simulink model "Main_Simulink"  (R2023b)
settings: Solver=FixedStepDiscrete  StartTime=0.0  StopTime=inf  FixedStep=0.001  RelTol=1e-3
undefined symbols (not defined in the file or in its folder): battery_builder_rtmsupport, gcbh, Initial_SOC
libraries: nesl_utility x118, pack_105s34p_structured_lib x105, fl_lib x14, ee_lib x7, dspstat3 x6, BatteryBalancing x1, deeplib x1
(part 2 of 10)

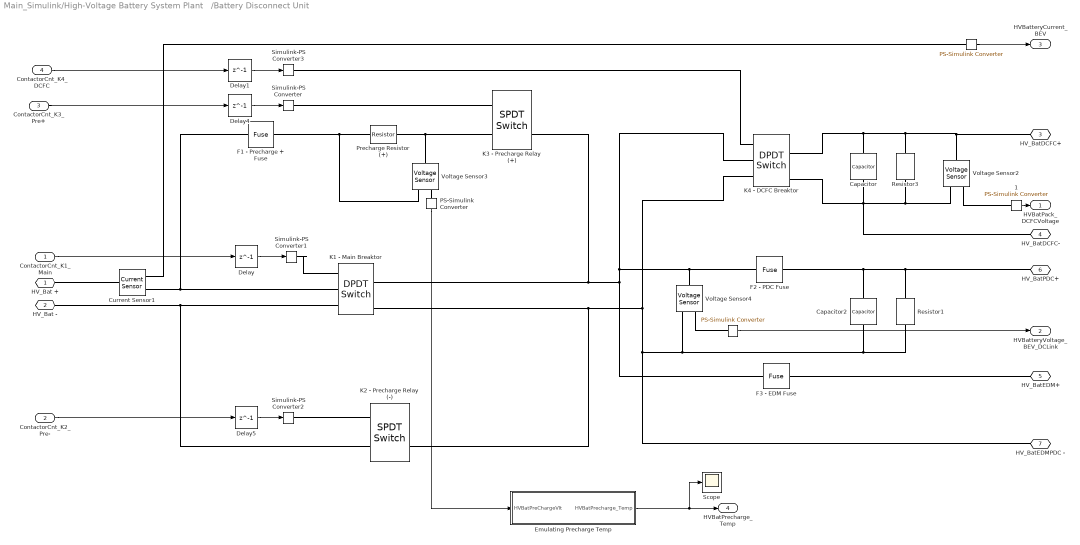
== system Main_Simulink/High-Voltage Battery System Plant   /Battery Disconnect Unit  ==
  ContactorCnt_K1_Main : Inport
  ContactorCnt_K2_Pre- : Inport  Port=2
  ContactorCnt_K3_Pre+ : Inport  Port=3
  ContactorCnt_K4_DCFC : Inport  Port=4
  "   " : nesl_utility/PS-Simulink Converter  PhysicalDomain=network_engine_domain  SubClassName=ps_output  LeftPortType=input  RightPortType=output  PseudoPeriodic=off  Frequencies=[]  VectorFormat=inherit  Unit=inherit  AffineConversion=off
  " " : nesl_utility/PS-Simulink Converter  PhysicalDomain=network_engine_domain  SubClassName=ps_output  LeftPortType=input  RightPortType=output  PseudoPeriodic=off  Frequencies=[]  VectorFormat=inherit  Unit=inherit  AffineConversion=off
  " 1" : nesl_utility/PS-Simulink Converter  PhysicalDomain=network_engine_domain  SubClassName=ps_output  LeftPortType=input  RightPortType=output  PseudoPeriodic=off  Frequencies=[]  VectorFormat=inherit  Unit=inherit  AffineConversion=off
  Capacitor : fl_lib/Electrical/Electrical Elements/Capacitor  c=750e-6 F  r=1e-6 Ohm  g=0 1/Ohm  i_specify=off  i_priority=None  i=0 A  i_nominal_specify=off  i_nominal_unit=A  i_nominal_value=1  v_specify=off  v_priority=None  v=0 V  v_nominal_specify=off  v_nominal_unit=V  v_nominal_value=1  vc_specify=off  vc_priority=High  vc=0 V  vc_nominal_specify=off  vc_nominal_unit=V  vc_nominal_value=1
  Capacitor2 : fl_lib/Electrical/Electrical Elements/Capacitor  c=750e-6 F  r=1e-6 Ohm  g=0 1/Ohm  i_specify=off  i_priority=None  i=0 A  i_nominal_specify=off  i_nominal_unit=A  i_nominal_value=1  v_specify=off  v_priority=None  v=0 V  v_nominal_specify=off  v_nominal_unit=V  v_nominal_value=1  vc_specify=off  vc_priority=High  vc=0 V  vc_nominal_specify=off  vc_nominal_unit=V  vc_nominal_value=1
  Current Sensor1 : fl_lib/Electrical/Electrical Sensors/Current Sensor
  Delay{,1,4..5} (4 alike) : Delay  DelayLength=1
  Emulating Precharge Temp : Subsystem
  F1 - Precharge + Fuse : ee_lib/Switches & Breakers/Fuse  prm=1  I_rated=600 A  melt_margin=1  T_fuse=0 s  I2t=1 A^2*s  I_vec=[1.9, 2, 2.5, 30] A  t_vec=[10000, 1, .3, .001] s  R_closed=0.01 Ohm  G_open=1e-8 1/Ohm  exposemeasurement=ee.enum.exposemeasurement.hidden
      settings: InternalSimscapePortConfiguration="{\"Bottom\":[],\"Left\":[{\"id\":\"p\",\"label\":\"\",\"type\":\"foundation.electrical.electrical\"}],\"Right\":[{\"id\":\"n\",\"label\":\"\",\"type\":\"foundation.electrical.electrical\"}],\"Top\":[]}"
  F2 - PDC Fuse : ee_lib/Switches & Breakers/Fuse  prm=1  I_rated=125 A  melt_margin=1  T_fuse=0 s  I2t=1 A^2*s  I_vec=[1.9, 2, 2.5, 30] A  t_vec=[10000, 1, .3, .001] s  R_closed=0.01 Ohm  G_open=1e-8 1/Ohm  exposemeasurement=ee.enum.exposemeasurement.hidden
      settings: InternalSimscapePortConfiguration="{\"Bottom\":[],\"Left\":[{\"id\":\"p\",\"label\":\"\",\"type\":\"foundation.electrical.electrical\"}],\"Right\":[{\"id\":\"n\",\"label\":\"\",\"type\":\"foundation.electrical.electrical\"}],\"Top\":[]}"
  F3 - EDM Fuse : ee_lib/Switches & Breakers/Fuse  prm=1  I_rated=600 A  melt_margin=1  T_fuse=0 s  I2t=1 A^2*s  I_vec=[1.9, 2, 2.5, 30] A  t_vec=[10000, 1, .3, .001] s  R_closed=0.01 Ohm  G_open=1e-8 1/Ohm  exposemeasurement=ee.enum.exposemeasurement.hidden
      settings: InternalSimscapePortConfiguration="{\"Bottom\":[],\"Left\":[{\"id\":\"p\",\"label\":\"\",\"type\":\"foundation.electrical.electrical\"}],\"Right\":[{\"id\":\"n\",\"label\":\"\",\"type\":\"foundation.electrical.electrical\"}],\"Top\":[]}"
  K1 - Main Breaktor : ee_lib/Switches & Breakers/DPDT Switch  R_closed=0.01 Ohm  G_open=1e-6 S  Threshold=0.5 V  Width=0 V  model_dynamics=0  t_on=1e-3 s  t_off=1e-3 s  initial_vT=0 V
      settings: InternalSimscapePortConfiguration="{\"Bottom\":[],\"Left\":[{\"id\":\"vT\",\"label\":\"vT\",\"type\":\"input\"},{\"id\":\"p1\",\"label\":\"\",\"type\":\"foundation.electrical.electrical\"},{\"id\":\"p2\",\"label\":\"\",\"type\":\"foundation.electrical.electrical\"}],\"Right\":[{\"id\":\"n11\",\"label\":\"\",\"type\":\"foundation.electrical.electrical\"},{\"id\":\"n12\",\"label\":\"\",\"type\":\"foundation.electrical.electrical\"},{\"id\":\"n21\",\"label\":\"\",\"type\":\"foundation.electrical.electrical\"},{\"id\":\"n22\",\"label\":\"\",\"type\":\"foundation.electrical.electrical\"}],\"Top\":[]}"
  K2 - Precharge Relay (-) : ee_lib/Switches & Breakers/SPDT Switch  R_closed=0.01 Ohm  G_open=1e-6 S  Threshold=0.5 V  Width=0 V  model_dynamics=0  t_on=1e-3 s  t_off=1e-3 s  initial_vT=0 V
  K3 - Precharge Relay (+) : ee_lib/Switches & Breakers/SPDT Switch  R_closed=0.01 Ohm  G_open=1e-6 S  Threshold=0.5 V  Width=0 V  model_dynamics=0  t_on=1e-3 s  t_off=1e-3 s  initial_vT=0 V
  K4 - DCFC Breaktor : ee_lib/Switches & Breakers/DPDT Switch  R_closed=0.01 Ohm  G_open=1e-6 S  Threshold=0.5 V  Width=0 V  model_dynamics=0  t_on=1e-3 s  t_off=1e-3 s  initial_vT=0 V
      settings: InternalSimscapePortConfiguration="{\"Bottom\":[],\"Left\":[{\"id\":\"vT\",\"label\":\"vT\",\"type\":\"input\"},{\"id\":\"p1\",\"label\":\"\",\"type\":\"foundation.electrical.electrical\"},{\"id\":\"p2\",\"label\":\"\",\"type\":\"foundation.electrical.electrical\"}],\"Right\":[{\"id\":\"n11\",\"label\":\"\",\"type\":\"foundation.electrical.electrical\"},{\"id\":\"n12\",\"label\":\"\",\"type\":\"foundation.electrical.electrical\"},{\"id\":\"n21\",\"label\":\"\",\"type\":\"foundation.electrical.electrical\"},{\"id\":\"n22\",\"label\":\"\",\"type\":\"foundation.electrical.electrical\"}],\"Top\":[]}"
  PS-Simulink Converter : nesl_utility/PS-Simulink Converter  PhysicalDomain=network_engine_domain  SubClassName=ps_output  LeftPortType=input  RightPortType=output  PseudoPeriodic=off  Frequencies=[]  VectorFormat=inherit  Unit=inherit  AffineConversion=off
  Precharge Resistor (+) : fl_lib/Electrical/Electrical Elements/Resistor  R=25 Ohm  i_specify=off  i_priority=None  i=0 A  i_nominal_specify=off  i_nominal_unit=A  i_nominal_value=1  v_specify=off  v_priority=None  v=0 V  v_nominal_specify=off  v_nominal_unit=V  v_nominal_value=1
  Resistor1 : fl_lib/Electrical/Electrical Elements/Resistor  R=40 kOhm  i_specify=off  i_priority=None  i=0 A  i_nominal_specify=off  i_nominal_unit=A  i_nominal_value=1  v_specify=off  v_priority=None  v=0 V  v_nominal_specify=off  v_nominal_unit=V  v_nominal_value=1
  Resistor3 : fl_lib/Electrical/Electrical Elements/Resistor  R=40 kOhm  i_specify=off  i_priority=None  i=0 A  i_nominal_specify=off  i_nominal_unit=A  i_nominal_value=1  v_specify=off  v_priority=None  v=0 V  v_nominal_specify=off  v_nominal_unit=V  v_nominal_value=1
  Scope : Scope
  Simulink-PS Converter{,1..3} (4 alike) : nesl_utility/Simulink-PS Converter  PhysicalDomain=network_engine_domain  SubClassName=ps_input  LeftPortType=input  RightPortType=output  PseudoPeriodic=off  Frequencies=[]  NoiseDistribution=none  NoiseParameters=[]  Unit=1  AffineConversion=off  FilteringAndDerivatives=provide  SimscapeFilterOrder=1  InputFilterTimeConstant=0.001  UdotUserProvided=0
  Voltage Sensor2 : fl_lib/Electrical/Electrical Sensors/Voltage Sensor
  Voltage Sensor3 : fl_lib/Electrical/Electrical Sensors/Voltage Sensor
  Voltage Sensor4 : fl_lib/Electrical/Electrical Sensors/Voltage Sensor
  "HV_Bat + " : PMIOPort  Side=Left
  HV_Bat - : PMIOPort  Port=2  Side=Left
  HV_BatDCFC+ : PMIOPort  Port=3  Side=Right
  HV_BatDCFC- : PMIOPort  Port=4  Side=Right
  HV_BatEDM+ : PMIOPort  Port=5  Side=Right
  HV_BatPDC+ : PMIOPort  Port=6  Side=Right
  HV_BatEDMPDC - : PMIOPort  Port=7  Side=Right
  HVBatPack_DCFCVoltage : Outport
  HVBatteryVoltage_BEV_DCLink : Outport  Port=2
  HVBatteryCurrent_BEV : Outport  Port=3
  HVBatPrecharge_Temp : Outport  Port=4
  wires:
  Delay1/1 -> Simulink-PS Converter3/1
  " 1"/1 -> HVBatPack_DCFCVoltage/1
  Delay5/1 -> Simulink-PS Converter2/1
  Delay4/1 -> Simulink-PS Converter/1
  "   "/1 -> HVBatteryCurrent_BEV/1
  ContactorCnt_K2_Pre-/1 -> Delay5/1
  Delay/1 -> Simulink-PS Converter1/1
  ContactorCnt_K4_DCFC/1 -> Delay1/1
  ContactorCnt_K1_Main/1 -> Delay/1
  ContactorCnt_K3_Pre+/1 -> Delay4/1
  PS-Simulink Converter/1 -> Emulating Precharge Temp/1(HVBatPreChargeVlt)
  " "/1 -> HVBatteryVoltage_BEV_DCLink/1
  Emulating Precharge Temp/1(HVBatPrecharge_Temp) -> Scope/1, HVBatPrecharge_Temp/1
  connections:
  Resistor3/LConn1 -- Voltage Sensor2/LConn1 -- HV_BatDCFC+/RConn1 -- Capacitor/LConn1 -- K4 - DCFC Breaktor/RConn2
  Voltage Sensor3/LConn1 -- K3 - Precharge Relay (+)/LConn2 -- Precharge Resistor (+)/LConn1
  Voltage Sensor3/RConn2 -- Precharge Resistor (+)/RConn1 -- F1 - Precharge + Fuse/RConn1
  Capacitor/RConn1 -- HV_BatDCFC-/RConn1 -- Voltage Sensor2/RConn2 -- Resistor3/RConn1 -- K4 - DCFC Breaktor/RConn4
  HV_BatEDM+/RConn1 -- F3 - EDM Fuse/LConn1
  Simulink-PS Converter1/RConn1 -- K1 - Main Breaktor/LConn1
  Voltage Sensor2/RConn1 -- " 1"/LConn1
  Resistor1/RConn1 -- Capacitor2/RConn1 -- HV_BatEDMPDC -/RConn1 -- K2 - Precharge Relay (-)/RConn2 -- K1 - Main Breaktor/RConn4 -- K4 - DCFC Breaktor/LConn3 -- Voltage Sensor4/RConn2
  "   "/LConn1 -- Current Sensor1/RConn1
  F2 - PDC Fuse/RConn1 -- Voltage Sensor4/LConn1 -- K3 - Precharge Relay (+)/RConn2 -- K1 - Main Breaktor/RConn2 -- F3 - EDM Fuse/RConn1 -- K4 - DCFC Breaktor/LConn2
  K2 - Precharge Relay (-)/LConn2 -- HV_Bat -/RConn1 -- K1 - Main Breaktor/LConn3
  K4 - DCFC Breaktor/LConn1 -- Simulink-PS Converter3/RConn1
  Simulink-PS Converter/RConn1 -- K3 - Precharge Relay (+)/LConn1
  Simulink-PS Converter2/RConn1 -- K2 - Precharge Relay (-)/LConn1
  F1 - Precharge + Fuse/LConn1 -- Current Sensor1/RConn2 -- K1 - Main Breaktor/LConn2
  PS-Simulink Converter/LConn1 -- Voltage Sensor3/RConn1
  Resistor1/LConn1 -- HV_BatPDC+/RConn1 -- F2 - PDC Fuse/LConn1 -- Capacitor2/LConn1
  Voltage Sensor4/RConn1 -- " "/LConn1
  "HV_Bat + "/RConn1 -- Current Sensor1/LConn1

== system Main_Simulink/High-Voltage Battery System Plant   /Charger//Load ==
  note: DC Fast Charging System
  note: Electric Drive Motor System
  note: Power Distribution Center System
  ChargeCurrentReq : Inport
  DrivingCurrentReq : Inport  Port=2
  ACChargeCurrentReq : Inport  Port=3
  Subsystem : Subsystem
  Subsystem1 : Subsystem
  Subsystem2 : Subsystem
  HV_BatDCFC+ : PMIOPort  Side=Left
  HV_BatDCFC- : PMIOPort  Port=2  Side=Left
  HV_BatEDM+ : PMIOPort  Port=3  Side=Left
  HV_BatPDC+ : PMIOPort  Port=4  Side=Left
  HV_BatEDMPDC - : PMIOPort  Port=5  Side=Left
  wires:
  ChargeCurrentReq/1 -> Subsystem/1(ChargeCurrentReq)
  DrivingCurrentReq/1 -> Subsystem1/1(DrivingCurrentReq)
  ACChargeCurrentReq/1 -> Subsystem2/1(ACChargeCurrentReq)
  connections:
  HV_BatDCFC+/RConn1 -- Subsystem/LConn1
  HV_BatDCFC-/RConn1 -- Subsystem/LConn2
  HV_BatEDMPDC -/RConn1 -- Subsystem2/LConn2 -- Subsystem1/LConn2
  HV_BatEDM+/RConn1 -- Subsystem1/LConn1
  HV_BatPDC+/RConn1 -- Subsystem2/LConn1

== system Main_Simulink/High-Voltage Battery System Plant   /ProMaster EV Battery Pack ==
  HVBatCellBalCmd : Inport
  Add : Sum
  Constant : Constant  Value=-273
  Constant1 : Constant  Value=25
  Constant2 : Constant  Value=25
  Delay : Delay  DelayLength=1
  Ground : fl_lib/Electrical/Electrical Elements/Electrical Reference
  "PS-Simulink " : nesl_utility/PS-Simulink Converter  PhysicalDomain=network_engine_domain  SubClassName=ps_output  LeftPortType=input  RightPortType=output  PseudoPeriodic=off  Frequencies=[]  VectorFormat=inherit  Unit=inherit  AffineConversion=off
  Pack1 : Subsystem  LoadFcn=battery_builder_rtmsupport('loadfcn',gcbh);
      settings: CopyFcn=battery_builder_rtmsupport('copyfcn',gcbh);  PreCopyFcn=battery_builder_rtmsupport('precopyfcn',gcbh);  PreDeleteFcn=battery_builder_rtmsupport('predeletefcn',gcbh);  PortSchema="{\"entries\":[{\"content\":{\"sides\":[{\"content\":{\"connectorIds\":[\"LConn1\"]},\"type\":\"ConnectorPlacement.EquallySpacedRectSide\",\"uuid\":\"64cec01f-33b3-4096-a4b7-6ded1472655c\"},{\"content\":{\"connectorIds\":[\"RConn1\"],\"side\":\"RIGHT\"},\"type\":\"ConnectorPlacement.EquallySpacedRectSide\",\"uuid\":\"f81a09ba-8909-4ce0-8a1f-4d13f5ea5620\"},{\"content\":{\"connectorIds\":[\"In1\"],\"side\":\"TOP\"},\"type\":\"ConnectorPlacement.EquallySpacedRectSide\",\"uuid\":\"a1cde63b-8eec-4d12-9d86-d553f5222491\"},{\"content\":{\"connectorIds\":[\"Out1\",\"Out2\",\"Out3\",\"Out4\",\"Out5\",\"Out6\",\"Out7\"],\"side\":\"BOTTOM\"},\"type\":\"ConnectorPlacement.EquallySpacedRectSide\",\"uuid\":\"7a252ceb-0eb8-4c98-af2a-dfdb6d4be7fd\"}]},\"type\":\"ConnectorPlacement.EquallySpacedConnector\",\"uuid\":\"c86ab74f-be26-4544-b601-79f59a4b6fde\"}],\"packageUris\":[\"http://schema.mathworks.com/mf0/Connector/R2020b\"],\"version\":\"1.0\"}"
      mask Display: image('$imagefile')
  Solver Configuration : nesl_utility/Solver Configuration  PhysicalDomain=network_engine_domain  SubClassName=solver  LeftPortType=input  RightPortType=generic  Tones=[]  Harmonics=[]  SimulateNoise=off  Profile=off  UseLocalSampling=off  EnableSwitchedLinearOptims=on  FrequencyDomain=off  UseCCode=off  RelTol=0.001  AbsTol=0.001  MinStep=1e-09  ToWorkspace=off  RevertToSquareIcSolve=off  NumHomotopyIterations=100  PhasorMode=off  PhasorModeNumHarmonics=1  ConsistencySolver=NEWTON_XTOL_AFTER_FTOL  IndexReductionMethod=DerivativeReplacement  DoDC=off  ResidualTolerance=1e-09  ConsistencyTolSource=GLOBAL  ConsistencyAbsTol=0.001  ConsistencyRelTol=0.001  ConsistencyTolFactor=0.001  UseLocalSolver=on  LocalSolverChoice=NE_BACKWARD_EULER_ADVANCER  ResolveIndetEquations=on  FunctionEvalNumThread=1  LocalSolverSampleTime=0.001  DoFixedCost=on  MaxNonlinIter=3  MaxModeIter=2  ComputeImpulses=off  ImpulseIterations=2  LinearAlgebra=auto  LinearAlgebraNumThread=0  EquationFormulation=NE_TIME_EF  DelaysMemoryBudget=1024  AutomaticFiltering=off  FilteringTimeConstant=0.001  PartitionStorageMethod=AS_NEEDED  PartitionMemoryBudget=1024  PartitionMethod=ROBUST  MultibodyUseLocalSolver=off  MultibodyLocalSolverChoice=ODE1  MultibodyLocalSolverSampleTime=0.001
  Terminator{1..5} (5 alike) : Terminator
  Voltage Sensor : fl_lib/Electrical/Electrical Sensors/Voltage Sensor
  "HV Bat + " : PMIOPort  Side=Right
  HV Bat - : PMIOPort  Port=2  Side=Right
  HVBatteryVoltage_BEV : Outport
  HVBatCellVlt : Outport  Port=2
  HVBatCellTemp : Outport  Port=3
  HVBatClgInletTemp : Outport  Port=4
  HVBatClgIOutletTemp : Outport  Port=5
  wires:
  Pack1/2(iCell) -> Terminator4/1
  Pack1/5(socParallelAssembly) -> Terminator2/1
  Pack1/1(vCell) -> HVBatCellVlt/1
  "PS-Simulink "/1 -> HVBatteryVoltage_BEV/1
  HVBatCellBalCmd/1 -> Delay/1
  Pack1/3(numCyclesCell) -> Terminator1/1
  Pack1/7(vParallelAssembly) -> Terminator3/1
  Delay/1 -> Pack1/1(balancing)
  Constant1/1 -> HVBatClgInletTemp/1
  Constant2/1 -> HVBatClgIOutletTemp/1
  Pack1/6(temperatureCell) -> Add/1
  Add/1 -> HVBatCellTemp/1
  Constant/1 -> Add/2
  Pack1/4(socCell) -> Terminator5/1
  connections:
  Voltage Sensor/RConn2 -- Ground/LConn1 -- Solver Configuration/RConn1 -- Pack1/RConn1 -- HV Bat -/RConn1
  "HV Bat + "/RConn1 -- Voltage Sensor/LConn1 -- Pack1/LConn1
  Voltage Sensor/RConn1 -- "PS-Simulink "/LConn1

== system Main_Simulink/Battery Management System/State of Charge Estimation System/Creating bus element ==
  HvBatSOCcell : Inport
  Bus Creator : BusCreator  Inputs=105
  Demux : Demux  Outputs=105
  HVBatSOCcell : Outport
  wires:
  Demux/23 -> Bus Creator/23
  Demux/82 -> Bus Creator/82
  Demux/22 -> Bus Creator/22
  Demux/30 -> Bus Creator/30
  Demux/75 -> Bus Creator/75
  Demux/13 -> Bus Creator/13
  Demux/66 -> Bus Creator/66
  Demux/31 -> Bus Creator/31
  Demux/12 -> Bus Creator/12
  Demux/56 -> Bus Creator/56
  Demux/27 -> Bus Creator/27
  Demux/64 -> Bus Creator/64
  Demux/86 -> Bus Creator/86
  Demux/100 -> Bus Creator/100
  Demux/89 -> Bus Creator/89
  Demux/90 -> Bus Creator/90
  Demux/94 -> Bus Creator/94
  Demux/101 -> Bus Creator/101
  Demux/91 -> Bus Creator/91
  Demux/96 -> Bus Creator/96
  Demux/97 -> Bus Creator/97
  Demux/105 -> Bus Creator/105
  Demux/104 -> Bus Creator/104
  Demux/84 -> Bus Creator/84
  Demux/85 -> Bus Creator/85
  Demux/80 -> Bus Creator/80
  Demux/83 -> Bus Creator/83
  Demux/21 -> Bus Creator/21
  Demux/42 -> Bus Creator/42
  Demux/74 -> Bus Creator/74
  Demux/95 -> Bus Creator/95
  Demux/41 -> Bus Creator/41
  Demux/102 -> Bus Creator/102
  Demux/14 -> Bus Creator/14
  Demux/7 -> Bus Creator/7
  Demux/63 -> Bus Creator/63
  Demux/20 -> Bus Creator/20
  Demux/78 -> Bus Creator/78
  Demux/87 -> Bus Creator/87
  Demux/59 -> Bus Creator/59
  Demux/26 -> Bus Creator/26
  Demux/33 -> Bus Creator/33
  Demux/32 -> Bus Creator/32
  Demux/73 -> Bus Creator/73
  Demux/28 -> Bus Creator/28
  Demux/15 -> Bus Creator/15
  Demux/17 -> Bus Creator/17
  Demux/35 -> Bus Creator/35
  Demux/93 -> Bus Creator/93
  Demux/16 -> Bus Creator/16
  Demux/29 -> Bus Creator/29
  Demux/71 -> Bus Creator/71
  Demux/47 -> Bus Creator/47
  Demux/19 -> Bus Creator/19
  Demux/10 -> Bus Creator/10
  Demux/54 -> Bus Creator/54
  Demux/18 -> Bus Creator/18
  Demux/53 -> Bus Creator/53
  Demux/11 -> Bus Creator/11
  Demux/81 -> Bus Creator/81
  Demux/70 -> Bus Creator/70
  Demux/3 -> Bus Creator/3
  Demux/52 -> Bus Creator/52
  Demux/5 -> Bus Creator/5
  Demux/1 -> Bus Creator/1
  Demux/37 -> Bus Creator/37
  Demux/68 -> Bus Creator/68
  Demux/38 -> Bus Creator/38
  Demux/8 -> Bus Creator/8
  Demux/58 -> Bus Creator/58
  Demux/34 -> Bus Creator/34
  Demux/103 -> Bus Creator/103
  Demux/98 -> Bus Creator/98
  Demux/24 -> Bus Creator/24
  Demux/36 -> Bus Creator/36
  Demux/62 -> Bus Creator/62
  Demux/39 -> Bus Creator/39
  Demux/88 -> Bus Creator/88
  Demux/40 -> Bus Creator/40
  Demux/50 -> Bus Creator/50
  Demux/92 -> Bus Creator/92
  Demux/55 -> Bus Creator/55
  Demux/43 -> Bus Creator/43
  Demux/48 -> Bus Creator/48
  Demux/60 -> Bus Creator/60
  Demux/49 -> Bus Creator/49
  Demux/25 -> Bus Creator/25
  Demux/57 -> Bus Creator/57
  Demux/45 -> Bus Creator/45
  Demux/46 -> Bus Creator/46
  Demux/69 -> Bus Creator/69
  Demux/67 -> Bus Creator/67
  Demux/65 -> Bus Creator/65
  Demux/9 -> Bus Creator/9
  Demux/61 -> Bus Creator/61
  Demux/99 -> Bus Creator/99
  Demux/76 -> Bus Creator/76
  Demux/72 -> Bus Creator/72
  Demux/6 -> Bus Creator/6
  Demux/77 -> Bus Creator/77
  Demux/4 -> Bus Creator/4
  Demux/79 -> Bus Creator/79
  Bus Creator/1 -> HVBatSOCcell/1
  HvBatSOCcell/1 -> Demux/1
  Demux/2 -> Bus Creator/2
  Demux/44 -> Bus Creator/44
  Demux/51 -> Bus Creator/51

== system Main_Simulink/Battery Management System/State of Charge Estimation System/For Each Subsystem1 ==
  HVBatteryCurrent_BEV : Inport
  HVBatCellVlt : Inport  Port=2  Partition=on  PartitionDimension=1  PartitionWidth=1  PartitionOffset=0
  HVBatCellTemp : Inport  Port=3  Partition=on  PartitionDimension=1  PartitionWidth=1  PartitionOffset=0
  Data Type Conversion : DataTypeConversion  SaturateOnIntegerOverflow=off  RndMeth=Floor
  Discrete Filter : DiscreteFilter  Numerator=[0.003131764229193,0.003131764229193]  Denominator=[1,-0.993736471541615]
  Discrete Filter1 : DiscreteFilter  Numerator=[0.003131764229193,0.003131764229193]  Denominator=[1,-0.993736471541615]
  Discrete Filter2 : DiscreteFilter  Numerator=[0.003131764229193,0.003131764229193]  Denominator=[1,-0.993736471541615]
  For Each : ForEach  DisableCoverage=on
  Gain : Gain  Gain=100
  MATLAB Function8 : MATLAB Function  TreatAsAtomicUnit=on
  Mux : Mux
  Normalize block - Current : Subsystem
  Normalize block - Kalman Filter SoC : Subsystem
  Normalize block - Temperature : Subsystem
  Normalize block -Voltage : Subsystem
  Predict : deeplib/Predict  Network=Network from MAT-file  NetworkFunction=squeezenet  NetworkFilePath=C:\Users\mcmas\Downloads\bwc\ProMaster RAM EV Plant\EKF-FNN.mat  MiniBatchSize=128  InputDataFormats={'',''}  Predictions=on  Activations={}  ForceInterpretedSim=off  EnableDLNetwork=on
      link override "MLFB/ Demux ": Outputs=1
      link override "MLFB/ SFunction ": FunctionName=sf_sfun
      link override MLFB/in_1: Port=1
      link override MLFB/out_1_predict: Port=1
  Subsystem : Subsystem
  Transpose{,1..3} (4 alike) : Math  Operator=transpose
  HvBatSOCcell : Outport  ConcatenationDimension=1
  wires:
  HVBatCellTemp/1 -> Subsystem/3(Temperature), Discrete Filter2/1
  Gain/1 -> HvBatSOCcell/1
  Discrete Filter1/1 -> Normalize block -Voltage/1(Voltage)
  Data Type Conversion/1 -> Gain/1
  Discrete Filter/1 -> Normalize block - Current/1(Current)
  Normalize block - Current/1(Normalized current) -> Transpose/1
  Transpose3/1 -> Mux/4
  Normalize block - Kalman Filter SoC/1(Normalized State of Charge) -> Transpose3/1
  Transpose/1 -> Mux/1
  Discrete Filter2/1 -> Normalize block - Temperature/1(Temperature)
  Transpose2/1 -> Mux/3
  Mux/1 -> Predict/1
  Subsystem/1(SOC) -> Normalize block - Kalman Filter SoC/1(State of Charge)
  Normalize block - Temperature/1(Normalized temperature) -> Transpose2/1
  Predict/1 -> MATLAB Function8/1(SOC)
  HVBatCellVlt/1 -> Subsystem/2(Voltage), Discrete Filter1/1
  Normalize block -Voltage/1(Normalized voltage) -> Transpose1/1
  HVBatteryCurrent_BEV/1 -> Subsystem/1(Current), Discrete Filter/1
  Transpose1/1 -> Mux/2
  MATLAB Function8/1(SOC_Output) -> Data Type Conversion/1

== system Main_Simulink/Battery Management System/State of Power Estimation System/Continuus Charge Power Limits ==
  note: Continuous Charge Power Limits
  note: Adjust to correct sign (Positive - Discharge; Negative - Charge)
  note: Convert to kW
  Bus Element In2 : Inport  PortName=BatteryMonitoringSystem  Element=HVBatteryCurrent_BEV
  Bus Element In3 : Inport  PortName=BatteryMonitoringSystem  Element=HVBatteryVoltage_BEV_Sec
  Bus Element In1 : Inport  Port=2  PortName=MaxPowerChrg  Element=Continuous
  Bus Element In4 : Inport  Port=2  PortName=MaxPowerChrg  Element=Instant
  Bus Element In5 : Inport  Port=2  PortName=MaxPowerChrg  Element=Short
  Bus Element In6 : Inport  Port=2  PortName=MaxPowerChrg  Element=Long
  Gain1 : Gain  Gain=-1
  Gain8 : Gain  Gain=1/1000
  MATLAB Function1 : MATLAB Function  TreatAsAtomicUnit=on  SystemSampleTime=1
  MATLAB Function3 : MATLAB Function  TreatAsAtomicUnit=on  SystemSampleTime=1
  MATLAB Function4 : MATLAB Function  TreatAsAtomicUnit=on  SystemSampleTime=1
  MATLAB Function5 : MATLAB Function  TreatAsAtomicUnit=on  SystemSampleTime=1
  Product : Product
  Terminator{1..4} (4 alike) : Terminator
  BPCM_HVBatChrgPowInstant : Outport
  BPCM_HVBatChrgPowShort : Outport  Port=2
  BPCM_HVBatChrgPowLong : Outport  Port=3
  BPCM_HVBatChrgPowCont : Outport  Port=4
  wires:
  Gain8/1 -> MATLAB Function5/1(Pt_kW)
  Gain1/1 -> Product/1
  Product/1 -> Gain8/1
  Bus Element In3/1 -> Product/2
  MATLAB Function5/4(E150_G) -> Terminator2/1
  MATLAB Function5/7(E180_G) -> Terminator4/1
  MATLAB Function5/6(E178_G) -> Terminator3/1
  MATLAB Function5/5(E170_G) -> Terminator1/1
  Bus Element In4/1 -> MATLAB Function1/1(P2_static)
  MATLAB Function5/1(P2_energy) -> MATLAB Function1/2(P2_energy)
  Bus Element In6/1 -> MATLAB Function4/1(P30_static)
  Bus Element In5/1 -> MATLAB Function3/1(P10_static)
  MATLAB Function5/2(P10_energy) -> MATLAB Function3/2(P10_energy)
  MATLAB Function5/3(P30_energy) -> MATLAB Function4/2(P30_energy)
  MATLAB Function1/1(P2_out) -> BPCM_HVBatChrgPowInstant/1
  MATLAB Function3/1(P10_out) -> BPCM_HVBatChrgPowShort/1
  MATLAB Function4/1(P30_out) -> BPCM_HVBatChrgPowLong/1
  Bus Element In1/1 -> MATLAB Function5/2(P180_kW), BPCM_HVBatChrgPowCont/1, MATLAB Function3/3(P180_kW), MATLAB Function1/3(P180_kW), MATLAB Function4/3(P180_kW)
  Bus Element In2/1 -> Gain1/1

== system Main_Simulink/Battery Management System/State of Power Estimation System/Continuus Discharge Power Limits ==
  note: Continuous Discharge Power Limits
  note: Adjust to correct sign (Positive - Discharge; Negative - Charge)
  note: Convert to kW
  Bus Element In1 : Inport  PortName=BatteryMonitoringSystem  Element=HVBatteryCurrent_BEV
  Bus Element In2 : Inport  PortName=BatteryMonitoringSystem  Element=HVBatteryVoltage_BEV_Sec
  Bus Element In3 : Inport  Port=2  PortName=MaxPowerDisch  Element=Continuous
  Bus Element In4 : Inport  Port=2  PortName=MaxPowerDisch  Element=Instant
  Bus Element In5 : Inport  Port=2  PortName=MaxPowerDisch  Element=Long
  Bus Element In6 : Inport  Port=2  PortName=MaxPowerDisch  Element=Short
  Gain1 : Gain  Gain=-1
  Gain8 : Gain  Gain=1/1000
  MATLAB Function1 : MATLAB Function  TreatAsAtomicUnit=on  SystemSampleTime=1
  MATLAB Function3 : MATLAB Function  TreatAsAtomicUnit=on  SystemSampleTime=1
  MATLAB Function4 : MATLAB Function  TreatAsAtomicUnit=on  SystemSampleTime=1
  MATLAB Function5 : MATLAB Function  TreatAsAtomicUnit=on  SystemSampleTime=1
  Product : Product
  Terminator{1..4} (4 alike) : Terminator
  BPCM_HVBatDischrgPowInstant : Outport
  BPCM_HVBatDischrgPowShort : Outport  Port=2
  BPCM_HVBatDischrgPowLong : Outport  Port=3
  BPCM_HVBatDischrgPowCont : Outport  Port=4
  wires:
  Gain8/1 -> MATLAB Function5/1(Pt_kW)
  Gain1/1 -> Product/1
  Product/1 -> Gain8/1
  Bus Element In2/1 -> Product/2
  Bus Element In1/1 -> Gain1/1
  MATLAB Function5/4(E150_G) -> Terminator2/1
  MATLAB Function5/7(E180_G) -> Terminator4/1
  MATLAB Function5/6(E178_G) -> Terminator3/1
  MATLAB Function5/5(E170_G) -> Terminator1/1
  Bus Element In4/1 -> MATLAB Function1/1(P2_static)
  MATLAB Function5/1(P2_energy) -> MATLAB Function1/2(P2_energy)
  Bus Element In5/1 -> MATLAB Function4/1(P30_static)
  Bus Element In6/1 -> MATLAB Function3/1(P10_static)
  MATLAB Function5/2(P10_energy) -> MATLAB Function3/2(P10_energy)
  MATLAB Function5/3(P30_energy) -> MATLAB Function4/2(P30_energy)
  MATLAB Function1/1(P2_out) -> BPCM_HVBatDischrgPowInstant/1
  MATLAB Function3/1(P10_out) -> BPCM_HVBatDischrgPowShort/1
  MATLAB Function4/1(P30_out) -> BPCM_HVBatDischrgPowLong/1
  Bus Element In3/1 -> MATLAB Function5/2(P180_kW), BPCM_HVBatDischrgPowCont/1, MATLAB Function3/3(P180_kW), MATLAB Function1/3(P180_kW), MATLAB Function4/3(P180_kW)

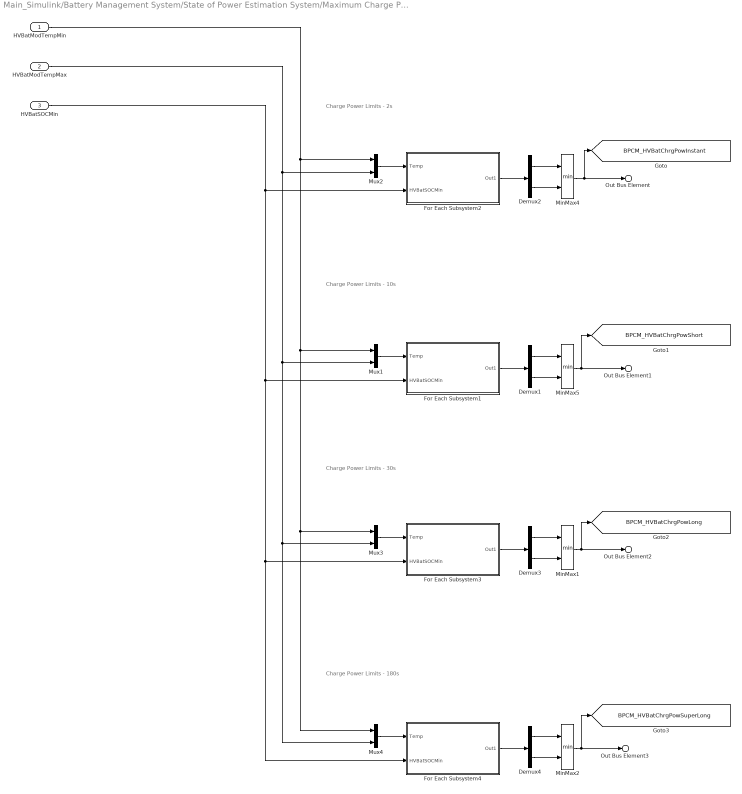
== system Main_Simulink/Battery Management System/State of Power Estimation System/Maximum Charge Power Limits ==
  note: Charge Power Limits - 180s
  note: Charge Power Limits - 30s
  note: Charge Power Limits - 10s
  note: Charge Power Limits - 2s
  HVBatModTempMin : Inport
  HVBatModTempMax : Inport  Port=2
  HVBatSOCMin : Inport  Port=3
  Demux{1..4} (4 alike) : Demux  Outputs=2
  For Each Subsystem1 : Subsystem  TreatAsAtomicUnit=on
  For Each Subsystem2 : Subsystem  TreatAsAtomicUnit=on
  For Each Subsystem3 : Subsystem  TreatAsAtomicUnit=on
  For Each Subsystem4 : Subsystem  TreatAsAtomicUnit=on
  MinMax{1..2,4..5} (4 alike) : MinMax  Inputs=2
  Mux{1..4} (4 alike) : Mux  Inputs=2
  Out Bus Element : Outport  PortName=MaxPowerChrg  Element=Instant
  Out Bus Element1 : Outport  PortName=MaxPowerChrg  Element=Short
  Out Bus Element2 : Outport  PortName=MaxPowerChrg  Element=Long
  Out Bus Element3 : Outport  PortName=MaxPowerChrg  Element=Continuous
  tag scope: BPCM_HVBatChrgPowInstant=global, BPCM_HVBatChrgPowLong=global, BPCM_HVBatChrgPowShort=global, BPCM_HVBatChrgPowSuperLong=global
  wires:
  Demux2/2 -> MinMax4/2
  MinMax4/1 -> [BPCM_HVBatChrgPowInstant], Out Bus Element/1
  Demux2/1 -> MinMax4/1
  For Each Subsystem2/1(Out1) -> Demux2/1
  Mux2/1 -> For Each Subsystem2/1(Temp)
  Demux1/2 -> MinMax5/2
  Demux1/1 -> MinMax5/1
  Mux1/1 -> For Each Subsystem1/1(Temp)
  For Each Subsystem1/1(Out1) -> Demux1/1
  MinMax5/1 -> Out Bus Element1/1, [BPCM_HVBatChrgPowShort]
  For Each Subsystem3/1(Out1) -> Demux3/1
  Mux3/1 -> For Each Subsystem3/1(Temp)
  Demux3/2 -> MinMax1/2
  Demux3/1 -> MinMax1/1
  MinMax1/1 -> Out Bus Element2/1, [BPCM_HVBatChrgPowLong]
  HVBatSOCMin/1 -> For Each Subsystem2/2(HVBatSOCMin), For Each Subsystem1/2(HVBatSOCMin), For Each Subsystem4/2(HVBatSOCMin), For Each Subsystem3/2(HVBatSOCMin)
  HVBatModTempMax/1 -> Mux4/2, Mux3/2, Mux1/2, Mux2/2
  Demux4/2 -> MinMax2/2
  Demux4/1 -> MinMax2/1
  For Each Subsystem4/1(Out1) -> Demux4/1
  Mux4/1 -> For Each Subsystem4/1(Temp)
  MinMax2/1 -> [BPCM_HVBatChrgPowSuperLong], Out Bus Element3/1
  HVBatModTempMin/1 -> Mux4/1, Mux3/1, Mux1/1, Mux2/1

== system Main_Simulink/Battery Management System/State of Power Estimation System/Maximum Discharge Power Limits ==
  note: Discharge Power Limits - 180s
  note: Discharge Power Limits - 30s
  note: Discharge Power Limits - 10s
  note: Discharge Power Limits - 2s
  HVBatModTempMin : Inport
  HVBatModTempMax : Inport  Port=2
  HVBatSOCMin : Inport  Port=3
  Demux{,1..3} (4 alike) : Demux  Outputs=2
  For Each Subsystem : Subsystem  TreatAsAtomicUnit=on
  For Each Subsystem1 : Subsystem  TreatAsAtomicUnit=on
  For Each Subsystem2 : Subsystem  TreatAsAtomicUnit=on
  For Each Subsystem3 : Subsystem  TreatAsAtomicUnit=on
  MinMax{1..4} (4 alike) : MinMax  Inputs=2
  Mux{,1..3} (4 alike) : Mux  Inputs=2
  Out Bus Element : Outport  PortName=MaxPowertDischg  Element=Instant
  Out Bus Element1 : Outport  PortName=MaxPowertDischg  Element=Short
  Out Bus Element2 : Outport  PortName=MaxPowertDischg  Element=Long
  Out Bus Element3 : Outport  PortName=MaxPowertDischg  Element=Continuous
  tag scope: BPCM_HVBatDischrgPowInstant=global, BPCM_HVBatDischrgPowLong=global, BPCM_HVBatDischrgPowShort=global, BPCM_HVBatDischrgPowSuperLong=global
  wires:
  Demux/1 -> MinMax4/1
  For Each Subsystem/1(Out1) -> Demux/1
  Demux/2 -> MinMax4/2
  Mux/1 -> For Each Subsystem/1(Temp)
  MinMax4/1 -> [BPCM_HVBatDischrgPowInstant], Out Bus Element/1
  Demux1/2 -> MinMax1/2
  Mux1/1 -> For Each Subsystem1/1(Temp)
  Demux1/1 -> MinMax1/1
  For Each Subsystem1/1(Out1) -> Demux1/1
  MinMax1/1 -> Out Bus Element1/1, [BPCM_HVBatDischrgPowShort]
  Demux2/1 -> MinMax2/1
  Mux2/1 -> For Each Subsystem2/1(Temp)
  HVBatModTempMax/1 -> Mux/2, Mux1/2, Mux3/2, Mux2/2
  Demux2/2 -> MinMax2/2
  HVBatModTempMin/1 -> Mux/1, Mux1/1, Mux3/1, Mux2/1
  For Each Subsystem2/1(Out1) -> Demux2/1
  MinMax2/1 -> Out Bus Element2/1, [BPCM_HVBatDischrgPowLong]
  Demux3/2 -> MinMax3/2
  MinMax3/1 -> Out Bus Element3/1, [BPCM_HVBatDischrgPowSuperLong]
  Demux3/1 -> MinMax3/1
  For Each Subsystem3/1(Out1) -> Demux3/1
  HVBatSOCMin/1 -> For Each Subsystem/2(HVBatSOCMin), For Each Subsystem1/2(HVBatSOCMin), For Each Subsystem2/2(HVBatSOCMin), For Each Subsystem3/2(HVBatSOCMin)
  Mux3/1 -> For Each Subsystem3/1(Temp)

== system Main_Simulink/High-Voltage Battery System Plant   /Battery Disconnect Unit /Emulating Precharge Temp ==
  note: Measuring precharge resistor temperature
      | 1. For every 100 ms, precharge relays are closed, at around 350 V, precharge resistor temperature increases by 4 degC,
      | 2. Assume initial precharge resistor temperature is 25 degC.
      | 3. If precharge resistr voltage is below 50 V, temperature doesn't increase.
  note: Input
      | precharge_resistor_voltage
      |
      | Output
      | precharge_resistor_temperature
  HVBatPreChargeVlt : Inport
  PrechargeResistorTemperature : MATLAB Function  TreatAsAtomicUnit=on
  HVBatPrecharge_Temp : Outport
  wires:
  HVBatPreChargeVlt/1 -> PrechargeResistorTemperature/1(V)
  PrechargeResistorTemperature/1(T) -> HVBatPrecharge_Temp/1

== system Main_Simulink/High-Voltage Battery System Plant   /Charger//Load/Subsystem ==
  ChargeCurrentReq : Inport
  Controlled Current Source : fl_lib/Electrical/Electrical Sources/Controlled Current Source
  Simulink-PS Converter4 : nesl_utility/Simulink-PS Converter  PhysicalDomain=network_engine_domain  SubClassName=ps_input  LeftPortType=input  RightPortType=output  PseudoPeriodic=off  Frequencies=[]  NoiseDistribution=none  NoiseParameters=[]  Unit=1  AffineConversion=off  FilteringAndDerivatives=provide  SimscapeFilterOrder=1  InputFilterTimeConstant=0.001  UdotUserProvided=0
  HV_BatDCFC+ : PMIOPort  Side=Left
  HV_BatDCFC- : PMIOPort  Port=2  Side=Left
  wires:
  ChargeCurrentReq/1 -> Simulink-PS Converter4/1
  connections:
  Simulink-PS Converter4/RConn1 -- Controlled Current Source/RConn1
  Controlled Current Source/LConn1 -- HV_BatDCFC+/RConn1
  Controlled Current Source/RConn2 -- HV_BatDCFC-/RConn1

== system Main_Simulink/High-Voltage Battery System Plant   /Charger//Load/Subsystem1 ==
  DrivingCurrentReq : Inport
  Controlled Current Source : fl_lib/Electrical/Electrical Sources/Controlled Current Source
  Simulink-PS Converter4 : nesl_utility/Simulink-PS Converter  PhysicalDomain=network_engine_domain  SubClassName=ps_input  LeftPortType=input  RightPortType=output  PseudoPeriodic=off  Frequencies=[]  NoiseDistribution=none  NoiseParameters=[]  Unit=1  AffineConversion=off  FilteringAndDerivatives=provide  SimscapeFilterOrder=1  InputFilterTimeConstant=0.001  UdotUserProvided=0
  HV_BatEDM+ : PMIOPort  Side=Left
  HV_BatEDMPDC - : PMIOPort  Port=2  Side=Left
  wires:
  DrivingCurrentReq/1 -> Simulink-PS Converter4/1
  connections:
  Simulink-PS Converter4/RConn1 -- Controlled Current Source/RConn1
  Controlled Current Source/LConn1 -- HV_BatEDM+/RConn1
  Controlled Current Source/RConn2 -- HV_BatEDMPDC -/RConn1

== system Main_Simulink/High-Voltage Battery System Plant   /Charger//Load/Subsystem2 ==
  ACChargeCurrentReq : Inport
  Controlled Current Source : fl_lib/Electrical/Electrical Sources/Controlled Current Source
  Simulink-PS Converter4 : nesl_utility/Simulink-PS Converter  PhysicalDomain=network_engine_domain  SubClassName=ps_input  LeftPortType=input  RightPortType=output  PseudoPeriodic=off  Frequencies=[]  NoiseDistribution=none  NoiseParameters=[]  Unit=1  AffineConversion=off  FilteringAndDerivatives=provide  SimscapeFilterOrder=1  InputFilterTimeConstant=0.001  UdotUserProvided=0
  HV_BatEDM+ : PMIOPort  Side=Left
  HV_BatEDMPDC - : PMIOPort  Port=2  Side=Left
  wires:
  ACChargeCurrentReq/1 -> Simulink-PS Converter4/1
  connections:
  Simulink-PS Converter4/RConn1 -- Controlled Current Source/RConn1
  Controlled Current Source/LConn1 -- HV_BatEDM+/RConn1
  Controlled Current Source/RConn2 -- HV_BatEDMPDC -/RConn1

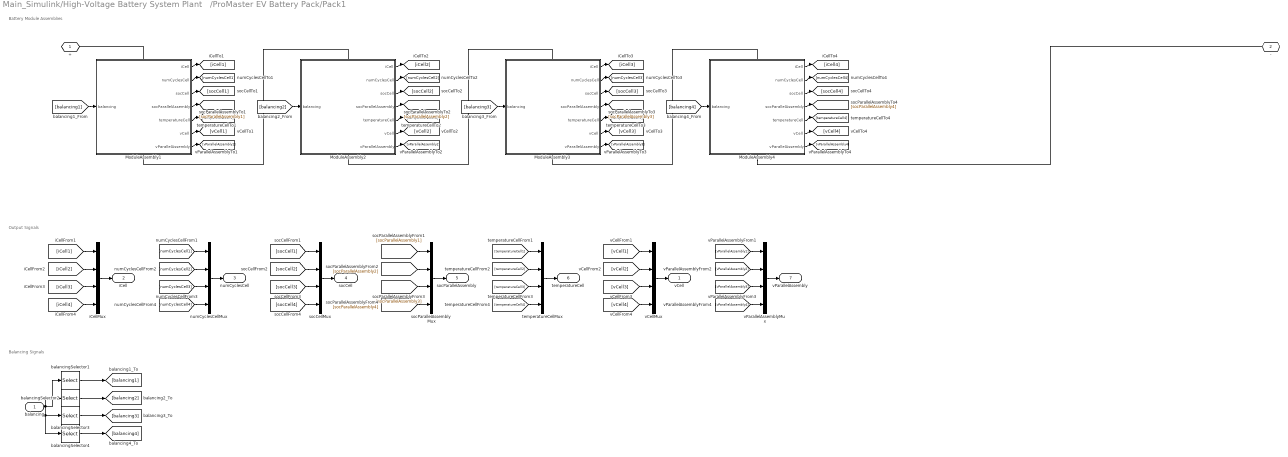
== system Main_Simulink/High-Voltage Battery System Plant   /ProMaster EV Battery Pack/Pack1 ==
  note: Battery Module Assemblies
  note: Output Signals
  note: Balancing Signals
  balancing : Inport  PortDimensions=105
  ModuleAssembly1 : Subsystem  LoadFcn=battery_builder_rtmsupport('loadfcn',gcbh);
      settings: CopyFcn=battery_builder_rtmsupport('copyfcn',gcbh);  PreCopyFcn=battery_builder_rtmsupport('precopyfcn',gcbh);  PreDeleteFcn=battery_builder_rtmsupport('predeletefcn',gcbh);  PortSchema="{\"entries\":[{\"content\":{\"sides\":[{\"content\":{\"connectorIds\":[\"LConn1\"]},\"type\":\"ConnectorPlacement.EquallySpacedRectSide\",\"uuid\":\"64cec01f-33b3-4096-a4b7-6ded1472655c\"},{\"content\":{\"connectorIds\":[\"RConn1\"],\"side\":\"RIGHT\"},\"type\":\"ConnectorPlacement.EquallySpacedRectSide\",\"uuid\":\"f81a09ba-8909-4ce0-8a1f-4d13f5ea5620\"},{\"content\":{\"connectorIds\":[\"In1\"],\"side\":\"TOP\"},\"type\":\"ConnectorPlacement.EquallySpacedRectSide\",\"uuid\":\"a1cde63b-8eec-4d12-9d86-d553f5222491\"},{\"content\":{\"connectorIds\":[\"Out1\",\"Out2\",\"Out3\",\"Out4\",\"Out5\",\"Out6\",\"Out7\"],\"side\":\"BOTTOM\"},\"type\":\"ConnectorPlacement.EquallySpacedRectSide\",\"uuid\":\"db89704a-c4ba-4090-9e93-a84dfb04aaf6\"}]},\"type\":\"ConnectorPlacement.EquallySpacedConnector\",\"uuid\":\"c86ab74f-be26-4544-b601-79f59a4b6fde\"}],\"packageUris\":[\"http://schema.mathworks.com/mf0/Connector/R2020b\"],\"version\":\"1.0\"}"
      mask Display: image('$imagefile')
  ModuleAssembly2 : Subsystem  LoadFcn=battery_builder_rtmsupport('loadfcn',gcbh);
      settings: CopyFcn=battery_builder_rtmsupport('copyfcn',gcbh);  PreCopyFcn=battery_builder_rtmsupport('precopyfcn',gcbh);  PreDeleteFcn=battery_builder_rtmsupport('predeletefcn',gcbh);  PortSchema="{\"entries\":[{\"content\":{\"sides\":[{\"content\":{\"connectorIds\":[\"LConn1\"]},\"type\":\"ConnectorPlacement.EquallySpacedRectSide\",\"uuid\":\"64cec01f-33b3-4096-a4b7-6ded1472655c\"},{\"content\":{\"connectorIds\":[\"RConn1\"],\"side\":\"RIGHT\"},\"type\":\"ConnectorPlacement.EquallySpacedRectSide\",\"uuid\":\"f81a09ba-8909-4ce0-8a1f-4d13f5ea5620\"},{\"content\":{\"connectorIds\":[\"In1\"],\"side\":\"TOP\"},\"type\":\"ConnectorPlacement.EquallySpacedRectSide\",\"uuid\":\"a1cde63b-8eec-4d12-9d86-d553f5222491\"},{\"content\":{\"connectorIds\":[\"Out1\",\"Out2\",\"Out3\",\"Out4\",\"Out5\",\"Out6\",\"Out7\"],\"side\":\"BOTTOM\"},\"type\":\"ConnectorPlacement.EquallySpacedRectSide\",\"uuid\":\"eef38c0f-4309-4f2b-bb03-9e449fb9f044\"}]},\"type\":\"ConnectorPlacement.EquallySpacedConnector\",\"uuid\":\"c86ab74f-be26-4544-b601-79f59a4b6fde\"}],\"packageUris\":[\"http://schema.mathworks.com/mf0/Connector/R2020b\"],\"version\":\"1.0\"}"
      mask Display: image('$imagefile')
  ModuleAssembly3 : Subsystem  LoadFcn=battery_builder_rtmsupport('loadfcn',gcbh);
      settings: CopyFcn=battery_builder_rtmsupport('copyfcn',gcbh);  PreCopyFcn=battery_builder_rtmsupport('precopyfcn',gcbh);  PreDeleteFcn=battery_builder_rtmsupport('predeletefcn',gcbh);  PortSchema="{\"entries\":[{\"content\":{\"sides\":[{\"content\":{\"connectorIds\":[\"LConn1\"]},\"type\":\"ConnectorPlacement.EquallySpacedRectSide\",\"uuid\":\"64cec01f-33b3-4096-a4b7-6ded1472655c\"},{\"content\":{\"connectorIds\":[\"RConn1\"],\"side\":\"RIGHT\"},\"type\":\"ConnectorPlacement.EquallySpacedRectSide\",\"uuid\":\"f81a09ba-8909-4ce0-8a1f-4d13f5ea5620\"},{\"content\":{\"connectorIds\":[\"In1\"],\"side\":\"TOP\"},\"type\":\"ConnectorPlacement.EquallySpacedRectSide\",\"uuid\":\"a1cde63b-8eec-4d12-9d86-d553f5222491\"},{\"content\":{\"connectorIds\":[\"Out1\",\"Out2\",\"Out3\",\"Out4\",\"Out5\",\"Out6\",\"Out7\"],\"side\":\"BOTTOM\"},\"type\":\"ConnectorPlacement.EquallySpacedRectSide\",\"uuid\":\"eef38c0f-4309-4f2b-bb03-9e449fb9f044\"}]},\"type\":\"ConnectorPlacement.EquallySpacedConnector\",\"uuid\":\"c86ab74f-be26-4544-b601-79f59a4b6fde\"}],\"packageUris\":[\"http://schema.mathworks.com/mf0/Connector/R2020b\"],\"version\":\"1.0\"}"
      mask Display: image('$imagefile')
  ModuleAssembly4 : Subsystem  LoadFcn=battery_builder_rtmsupport('loadfcn',gcbh);
      settings: CopyFcn=battery_builder_rtmsupport('copyfcn',gcbh);  PreCopyFcn=battery_builder_rtmsupport('precopyfcn',gcbh);  PreDeleteFcn=battery_builder_rtmsupport('predeletefcn',gcbh);  PortSchema="{\"entries\":[{\"content\":{\"sides\":[{\"content\":{\"connectorIds\":[\"LConn1\"]},\"type\":\"ConnectorPlacement.EquallySpacedRectSide\",\"uuid\":\"64cec01f-33b3-4096-a4b7-6ded1472655c\"},{\"content\":{\"connectorIds\":[\"RConn1\"],\"side\":\"RIGHT\"},\"type\":\"ConnectorPlacement.EquallySpacedRectSide\",\"uuid\":\"f81a09ba-8909-4ce0-8a1f-4d13f5ea5620\"},{\"content\":{\"connectorIds\":[\"In1\"],\"side\":\"TOP\"},\"type\":\"ConnectorPlacement.EquallySpacedRectSide\",\"uuid\":\"a1cde63b-8eec-4d12-9d86-d553f5222491\"},{\"content\":{\"connectorIds\":[\"Out1\",\"Out2\",\"Out3\",\"Out4\",\"Out5\",\"Out6\",\"Out7\"],\"side\":\"BOTTOM\"},\"type\":\"ConnectorPlacement.EquallySpacedRectSide\",\"uuid\":\"eef38c0f-4309-4f2b-bb03-9e449fb9f044\"}]},\"type\":\"ConnectorPlacement.EquallySpacedConnector\",\"uuid\":\"c86ab74f-be26-4544-b601-79f59a4b6fde\"}],\"packageUris\":[\"http://schema.mathworks.com/mf0/Connector/R2020b\"],\"version\":\"1.0\"}"
      mask Display: image('$imagefile')
  balancingSelector1 : Selector  InputPortWidth=105  IndexOptions=Index vector (dialog)  Indices="[1   2   3   4   5   6   7   8   9  10  11  12  13  14  15  16  17  18  19  20  21  22  23  24]"  OutputSizes=1
  balancingSelector2 : Selector  InputPortWidth=105  IndexOptions=Index vector (dialog)  Indices="[25  26  27  28  29  30  31  32  33  34  35  36  37  38  39  40  41  42  43  44  45  46  47  48  49  50  51]"  OutputSizes=1
  balancingSelector3 : Selector  InputPortWidth=105  IndexOptions=Index vector (dialog)  Indices="[52  53  54  55  56  57  58  59  60  61  62  63  64  65  66  67  68  69  70  71  72  73  74  75  76  77  78]"  OutputSizes=1
  balancingSelector4 : Selector  InputPortWidth=105  IndexOptions=Index vector (dialog)  Indices="[79   80   81   82   83   84   85   86   87   88   89   90   91   92   93   94   95   96   97   98   99  100  101  102  103  104  105]"  OutputSizes=1
  iCellMux : Mux
  numCyclesCellMux : Mux
  socCellMux : Mux
  socParallelAssemblyMux : Mux
  temperatureCellMux : Mux
  vCellMux : Mux
  vParallelAssemblyMux : Mux
  + : PMIOPort  Side=Left
  - : PMIOPort  Port=2  Side=Right
  vCell : Outport
  iCell : Outport  Port=2
  numCyclesCell : Outport  Port=3
  socCell : Outport  Port=4
  socParallelAssembly : Outport  Port=5
  temperatureCell : Outport  Port=6
  vParallelAssembly : Outport  Port=7
  wires:
  ModuleAssembly1/1(iCell) -> [iCell1]
  iCellMux/1 -> iCell/1
  [iCell1] -> iCellMux/1
  ModuleAssembly1/2(numCyclesCell) -> [numCyclesCell1]
  numCyclesCellMux/1 -> numCyclesCell/1
  [numCyclesCell1] -> numCyclesCellMux/1
  ModuleAssembly1/3(socCell) -> [socCell1]
  socCellMux/1 -> socCell/1
  [socCell1] -> socCellMux/1
  ModuleAssembly1/4(socParallelAssembly) -> [socParallelAssembly1]
  socParallelAssemblyMux/1 -> socParallelAssembly/1
  [socParallelAssembly1] -> socParallelAssemblyMux/1
  ModuleAssembly1/5(temperatureCell) -> [temperatureCell1]
  temperatureCellMux/1 -> temperatureCell/1
  [temperatureCell1] -> temperatureCellMux/1
  ModuleAssembly1/6(vCell) -> [vCell1]
  vCellMux/1 -> vCell/1
  [vCell1] -> vCellMux/1
  ModuleAssembly1/7(vParallelAssembly) -> [vParallelAssembly1]
  vParallelAssemblyMux/1 -> vParallelAssembly/1
  [vParallelAssembly1] -> vParallelAssemblyMux/1
  ModuleAssembly2/1(iCell) -> [iCell2]
  [iCell2] -> iCellMux/2
  ModuleAssembly2/2(numCyclesCell) -> [numCyclesCell2]
  [numCyclesCell2] -> numCyclesCellMux/2
  ModuleAssembly2/3(socCell) -> [socCell2]
  [socCell2] -> socCellMux/2
  ModuleAssembly2/4(socParallelAssembly) -> [socParallelAssembly2]
  [socParallelAssembly2] -> socParallelAssemblyMux/2
  ModuleAssembly2/5(temperatureCell) -> [temperatureCell2]
  [temperatureCell2] -> temperatureCellMux/2
  ModuleAssembly2/6(vCell) -> [vCell2]
  [vCell2] -> vCellMux/2
  ModuleAssembly2/7(vParallelAssembly) -> [vParallelAssembly2]
  [vParallelAssembly2] -> vParallelAssemblyMux/2
  ModuleAssembly3/1(iCell) -> [iCell3]
  [iCell3] -> iCellMux/3
  ModuleAssembly3/2(numCyclesCell) -> [numCyclesCell3]
  [numCyclesCell3] -> numCyclesCellMux/3
  ModuleAssembly3/3(socCell) -> [socCell3]
  [socCell3] -> socCellMux/3
  ModuleAssembly3/4(socParallelAssembly) -> [socParallelAssembly3]
  [socParallelAssembly3] -> socParallelAssemblyMux/3
  ModuleAssembly3/5(temperatureCell) -> [temperatureCell3]
  [temperatureCell3] -> temperatureCellMux/3
  ModuleAssembly3/6(vCell) -> [vCell3]
  [vCell3] -> vCellMux/3
  ModuleAssembly3/7(vParallelAssembly) -> [vParallelAssembly3]
  [vParallelAssembly3] -> vParallelAssemblyMux/3
  ModuleAssembly4/1(iCell) -> [iCell4]
  [iCell4] -> iCellMux/4
  ModuleAssembly4/2(numCyclesCell) -> [numCyclesCell4]
  [numCyclesCell4] -> numCyclesCellMux/4
  ModuleAssembly4/3(socCell) -> [socCell4]
  [socCell4] -> socCellMux/4
  ModuleAssembly4/4(socParallelAssembly) -> [socParallelAssembly4]
  [socParallelAssembly4] -> socParallelAssemblyMux/4
  ModuleAssembly4/5(temperatureCell) -> [temperatureCell4]
  [temperatureCell4] -> temperatureCellMux/4
  ModuleAssembly4/6(vCell) -> [vCell4]
  [vCell4] -> vCellMux/4
  ModuleAssembly4/7(vParallelAssembly) -> [vParallelAssembly4]
  [vParallelAssembly4] -> vParallelAssemblyMux/4
  [balancing1] -> ModuleAssembly1/1(balancing)
  balancing/1 -> balancingSelector3/1, balancingSelector4/1, balancingSelector1/1, balancingSelector2/1
  balancingSelector1/1 -> [balancing1]
  [balancing2] -> ModuleAssembly2/1(balancing)
  balancingSelector2/1 -> [balancing2]
  [balancing3] -> ModuleAssembly3/1(balancing)
  balancingSelector3/1 -> [balancing3]
  [balancing4] -> ModuleAssembly4/1(balancing)
  balancingSelector4/1 -> [balancing4]
  connections:
  ModuleAssembly2/LConn1 -- ModuleAssembly1/RConn1
  ModuleAssembly3/LConn1 -- ModuleAssembly2/RConn1
  ModuleAssembly4/LConn1 -- ModuleAssembly3/RConn1
  ModuleAssembly1/LConn1 -- +/RConn1
  ModuleAssembly4/RConn1 -- -/RConn1

== system Main_Simulink/Battery Management System/State of Charge Estimation System/For Each Subsystem1/Normalize block - Current ==
  note: McMaster Automotive Research Centre (MARC)
      | Electrical Engineer - Romulo Navega Vieira - M.Sc and MBA - PhD Candidate
  Current : Inport
  Constant : Constant  Value=-7.4943
  Constant1 : Constant  Value=-7.4943
  Constant2 : Constant  Value=6.2959
  Divide : Product  Inputs=*/
  Sum : Sum  Inputs=|+-
  Sum1 : Sum  Inputs=|+-
  Normalized current : Outport
  wires:
  Current/1 -> Sum/1
  Sum/1 -> Divide/1
  Sum1/1 -> Divide/2
  Divide/1 -> Normalized current/1
  Constant/1 -> Sum/2
  Constant2/1 -> Sum1/1
  Constant1/1 -> Sum1/2

== system Main_Simulink/Battery Management System/State of Charge Estimation System/For Each Subsystem1/Normalize block - Kalman Filter SoC ==
  note: McMaster Automotive Research Centre (MARC)
      | Electrical Engineer - Romulo Navega Vieira - M.Sc and MBA - PhD Candidate
  State of Charge : Inport
  Constant : Constant  Value=0
  Constant1 : Constant  Value=0
  Constant2 : Constant
  Divide : Product  Inputs=*/
  Sum : Sum  Inputs=|+-
  Sum1 : Sum  Inputs=|+-
  Normalized State of Charge : Outport
  wires:
  State of Charge/1 -> Sum/1
  Sum/1 -> Divide/1
  Sum1/1 -> Divide/2
  Divide/1 -> Normalized State of Charge/1
  Constant/1 -> Sum/2
  Constant2/1 -> Sum1/1
  Constant1/1 -> Sum1/2

== system Main_Simulink/Battery Management System/State of Charge Estimation System/For Each Subsystem1/Normalize block - Temperature ==
  note: McMaster Automotive Research Centre (MARC)
      | Electrical Engineer - Romulo Navega Vieira - M.Sc and MBA - PhD Candidate
  Temperature : Inport
  Constant : Constant  Value=-20.8609
  Constant1 : Constant  Value=-20.8609
  Constant2 : Constant  Value=40.3838
  Divide : Product  Inputs=*/
  Sum : Sum  Inputs=|+-
  Sum1 : Sum  Inputs=|+-
  Normalized temperature : Outport
  wires:
  Temperature/1 -> Sum/1
  Sum/1 -> Divide/1
  Sum1/1 -> Divide/2
  Divide/1 -> Normalized temperature/1
  Constant/1 -> Sum/2
  Constant2/1 -> Sum1/1
  Constant1/1 -> Sum1/2

== system Main_Simulink/Battery Management System/State of Charge Estimation System/For Each Subsystem1/Normalize block -Voltage ==
  note: McMaster Automotive Research Centre (MARC)
      | Electrical Engineer - Romulo Navega Vieira - M.Sc and MBA - PhD Candidate
  Voltage : Inport
  Constant : Constant  Value=2.7108
  Constant1 : Constant  Value=2.7108
  Constant2 : Constant  Value=4.3838
  Divide : Product  Inputs=*/
  Sum : Sum  Inputs=|+-
  Sum1 : Sum  Inputs=|+-
  Normalized voltage : Outport
  wires:
  Voltage/1 -> Sum/1
  Sum/1 -> Divide/1
  Sum1/1 -> Divide/2
  Divide/1 -> Normalized voltage/1
  Constant/1 -> Sum/2
  Constant2/1 -> Sum1/1
  Constant1/1 -> Sum1/2

== system Main_Simulink/Battery Management System/State of Charge Estimation System/For Each Subsystem1/Subsystem ==
  note: McMaster Automotive Research Centre - MARC
      | Electrical Engineer: Romulo Navega Vieira, M.Sc and MBA - PhD Candidate
  Current : Inport
  Voltage : Inport  Port=2
  Temperature : Inport  Port=3
  Constant1 : Constant  Value=[0;0;0]
  Delay2 : Delay  DelayLength=1  InitialConditionSource=Input port  InitialCondition=[0;0;0;Initial_SOC]
      settings: InputPortMap=u0,p4
  Delay3 : Delay  DelayLength=1  InitialCondition=diag([1 1 1 0.01])
  Equivalent Circuit Model : Subsystem
  Extended Kalman Filter : MATLAB Function  TreatAsAtomicUnit=on
  Saturation : Saturate  UpperLimit=1  LowerLimit=0
  Subsystem : Subsystem
  Vector Concatenate : Concatenate
  SOC : Outport
  wires:
  Subsystem/4(Q3) -> Extended Kalman Filter/16(Q3)
  Equivalent Circuit Model/5(R3Prime) -> Extended Kalman Filter/9(R3)
  Equivalent Circuit Model/9(Capacity Ah) -> Extended Kalman Filter/18(Capacity_Ah)
  Subsystem/5(Q4) -> Extended Kalman Filter/17(Q4)
  Voltage/1 -> Equivalent Circuit Model/3(Initial Voltage), Extended Kalman Filter/2(Voltage)
  Equivalent Circuit Model/7(C2Prime) -> Extended Kalman Filter/11(C2)
  Vector Concatenate/1 -> Delay2/2
  Delay3/1 -> Extended Kalman Filter/5(P)
  Extended Kalman Filter/2(xf) -> Delay2/1
  Equivalent Circuit Model/2(R0Prime) -> Extended Kalman Filter/6(R0)
  Extended Kalman Filter/1(zSOC) -> Saturation/1
  Temperature/1 -> Extended Kalman Filter/3(Temperature), Subsystem/1(Temeperature), Equivalent Circuit Model/2(Temperature)
  Equivalent Circuit Model/1(Initial SOC) -> Vector Concatenate/2
  Subsystem/1(R) -> Extended Kalman Filter/13(R)
  Subsystem/3(Q2) -> Extended Kalman Filter/15(Q2)
  Constant1/1 -> Vector Concatenate/1
  Subsystem/2(Q1) -> Extended Kalman Filter/14(Q1)
  Delay2/1 -> Extended Kalman Filter/4(x)
  Extended Kalman Filter/3(P1) -> Delay3/1
  Saturation/1 -> SOC/1, Equivalent Circuit Model/1(State of Charge)
  Equivalent Circuit Model/6(C1Prime) -> Extended Kalman Filter/10(C1)
  Equivalent Circuit Model/8(C3Prime) -> Extended Kalman Filter/12(C3)
  Equivalent Circuit Model/4(R2Prime) -> Extended Kalman Filter/8(R2)
  Current/1 -> Extended Kalman Filter/1(Current)
  Equivalent Circuit Model/3(R1Prime) -> Extended Kalman Filter/7(R1)
